simulink model "GhendyanoT2F"  (R2021b)
settings: Solver=ode45  StartTime=0.0  StopTime=TempoSimulacao  RelTol=1e-3  EnableMultiTasking=on
values from neighbouring files (symbols this model uses):
  ccc1 = Ccc*d    [TesteRealCurtoFuses.m]    (also in TesteRealCurto_SemFuse.m)
  ccc2 = Ccc*d    [TesteRealCurtoFuses.m]    (also in TesteRealCurto_SemFuse.m)
  cct1 = Cct*d    [TesteRealCurtoFuses.m]    (also in TesteRealCurto_SemFuse.m)
  cct2 = Cct*d    [TesteRealCurtoFuses.m]    (also in TesteRealCurto_SemFuse.m)
  cequa1 = Ceq*d    [TesteRealCurtoFuses.m]    (also in TesteRealCurto_SemFuse.m)
  cequa2 = Ceq*d    [TesteRealCurtoFuses.m]    (also in TesteRealCurto_SemFuse.m)
  FatorSimulacao = 1e-3    (= 0.001)    [TesteRealCurtoFuses.m]    (also in TesteRealCurto_SemFuse.m)
  le = 1e-10    [TesteRealCurto.m]    (also in TesteRealCurtoFuses.m; TesteRealCurto_SemFuse.m)
  lm1 = lm    [TesteRealCurto.m]    (also in TesteRealCurtoFuses.m; TesteRealCurto_SemFuse.m)
  lm2 = lm    [TesteRealCurto.m]    (also in TesteRealCurtoFuses.m; TesteRealCurto_SemFuse.m)
  lp1 = lp    [TesteRealCurto.m]    (also in TesteRealCurtoFuses.m; TesteRealCurto_SemFuse.m)
  lp2 = lp    [TesteRealCurto.m]    (also in TesteRealCurtoFuses.m; TesteRealCurto_SemFuse.m)
  NRE = 1e-12    [TesteRealCurto.m]    (also in TesteRealCurtoFuses.m; TesteRealCurto_SemFuse.m)
  Raf1 = inf    [TesteRealCurto.m]    (also in TesteRealCurtoFuses.m; TesteRealCurto_SemFuse.m)
  Raf2 = inf    [TesteRealCurto.m]    (also in TesteRealCurtoFuses.m; TesteRealCurto_SemFuse.m)
  Rbf1 = inf    [TesteRealCurto.m]    (also in TesteRealCurtoFuses.m; TesteRealCurto_SemFuse.m)
  Rbf2 = inf    [TesteRealCurto.m]    (also in TesteRealCurtoFuses.m; TesteRealCurto_SemFuse.m)
  Rcf1 = inf    [TesteRealCurto.m]    (also in TesteRealCurtoFuses.m; TesteRealCurto_SemFuse.m)
  Rcf2 = inf    [TesteRealCurto.m]    (also in TesteRealCurtoFuses.m; TesteRealCurto_SemFuse.m)
  rm1 = rm    [TesteRealCurto.m]    (also in TesteRealCurtoFuses.m; TesteRealCurto_SemFuse.m)
  rm2 = rm    [TesteRealCurto.m]    (also in TesteRealCurtoFuses.m; TesteRealCurto_SemFuse.m)
  rp1 = rp    [TesteRealCurto.m]    (also in TesteRealCurtoFuses.m; TesteRealCurto_SemFuse.m)
  rp2 = rp    [TesteRealCurto.m]    (also in TesteRealCurtoFuses.m; TesteRealCurto_SemFuse.m)
  rtc1 = 8    [TesteRealCurto.m]    (also in TesteRealCurtoFuses.m; TesteRealCurto_SemFuse.m)
  rtc2 = 8    [TesteRealCurto.m]    (also in TesteRealCurtoFuses.m; TesteRealCurto_SemFuse.m)
  rti = 10    [TesteRealCurto.m]    (also in TesteRealCurtoFuses.m; TesteRealCurto_SemFuse.m)
undefined symbols (not defined in the file or in its folder): D11, Delta
libraries: spsSeriesRLCBranchLib x26, spsRMSLib x14, spsBreakerLib x9, spsCurrentMeasurementLib x9, spsThreePhaseTransformerTwoWindingsLib x4, spsThreePhaseVIMeasurementLib x3, spsMutualInductanceLib x2, spsThreePhaseSeriesRLCLoadLib x2, spsThreePhaseSourceLib x1, spspowerguiLib x1
(part 2 of 2)

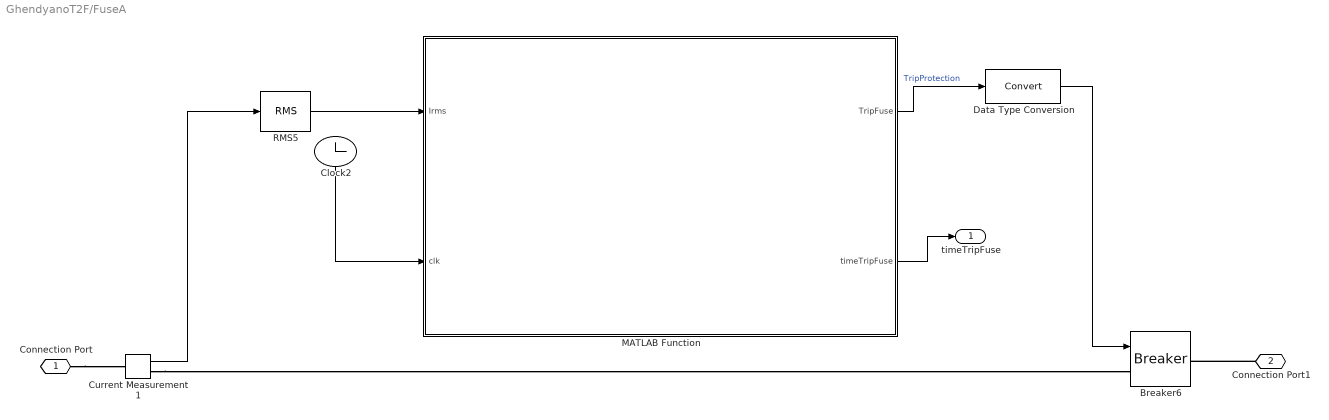
== system GhendyanoT2F/FuseA ==
  Breaker6 : spsBreakerLib/Breaker  InitialState=1  SwitchingTimes="[1/60  5/60]"  External=on  BreakerResistance=0.01  SnubberResistance=1e6  SnubberCapacitance=inf  Measurements=None  MoreParameters=on  NoBreakLoop=off
      settings: SourceProductBaseCode=PS
  Clock2 : Clock
      settings: Decimation=1000
  Current Measurement1 : spsCurrentMeasurementLib/Current Measurement  PhasorSimulation=off  OutputType=Complex  PSBequivalent=0
  Data Type Conversion : DataTypeConversion
  MATLAB Function : MATLAB Function
  RMS5 : spsRMSLib/RMS  TrueRMS=on  Freq=60  RMSInit=0  Ts=0
  Connection Port : PMIOPort  Side=Right
  Connection Port1 : PMIOPort  Port=2  Side=Left
  timeTripFuse : Outport
  wires:
  MATLAB Function/1(TripFuse) -> Data Type Conversion/1  "TripProtection"
  RMS5/1 -> MATLAB Function/1(Irms)
  Data Type Conversion/1 -> Breaker6/1
  Current Measurement1/1 -> RMS5/1
  Clock2/1 -> MATLAB Function/2(clk)
  MATLAB Function/2(timeTripFuse) -> timeTripFuse/1
  connections:
  Current Measurement1/RConn1 -- Breaker6/LConn1
  Connection Port/RConn1 -- Current Measurement1/LConn1
  Connection Port1/RConn1 -- Breaker6/RConn1

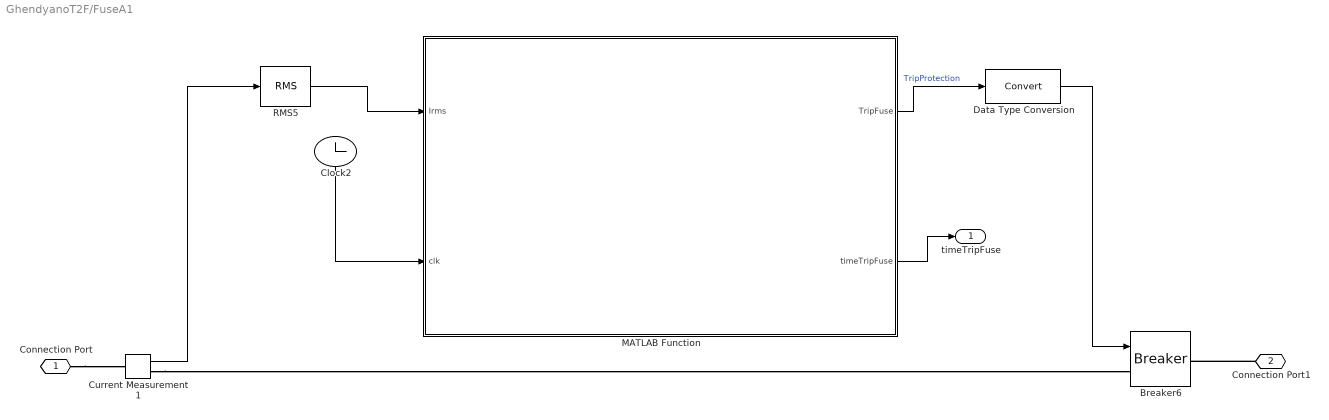
== system GhendyanoT2F/FuseA1 ==
  Breaker6 : spsBreakerLib/Breaker  InitialState=1  SwitchingTimes="[1/60  5/60]"  External=on  BreakerResistance=0.01  SnubberResistance=1e6  SnubberCapacitance=inf  Measurements=None  MoreParameters=on  NoBreakLoop=off
      settings: SourceProductBaseCode=PS
  Clock2 : Clock
      settings: Decimation=1000
  Current Measurement1 : spsCurrentMeasurementLib/Current Measurement  PhasorSimulation=off  OutputType=Complex  PSBequivalent=0
  Data Type Conversion : DataTypeConversion
  MATLAB Function : MATLAB Function
  RMS5 : spsRMSLib/RMS  TrueRMS=on  Freq=60  RMSInit=0  Ts=0
  Connection Port : PMIOPort  Side=Right
  Connection Port1 : PMIOPort  Port=2  Side=Left
  timeTripFuse : Outport
  wires:
  MATLAB Function/1(TripFuse) -> Data Type Conversion/1  "TripProtection"
  RMS5/1 -> MATLAB Function/1(Irms)
  Data Type Conversion/1 -> Breaker6/1
  Current Measurement1/1 -> RMS5/1
  Clock2/1 -> MATLAB Function/2(clk)
  MATLAB Function/2(timeTripFuse) -> timeTripFuse/1
  connections:
  Current Measurement1/RConn1 -- Breaker6/LConn1
  Connection Port/RConn1 -- Current Measurement1/LConn1
  Connection Port1/RConn1 -- Breaker6/RConn1

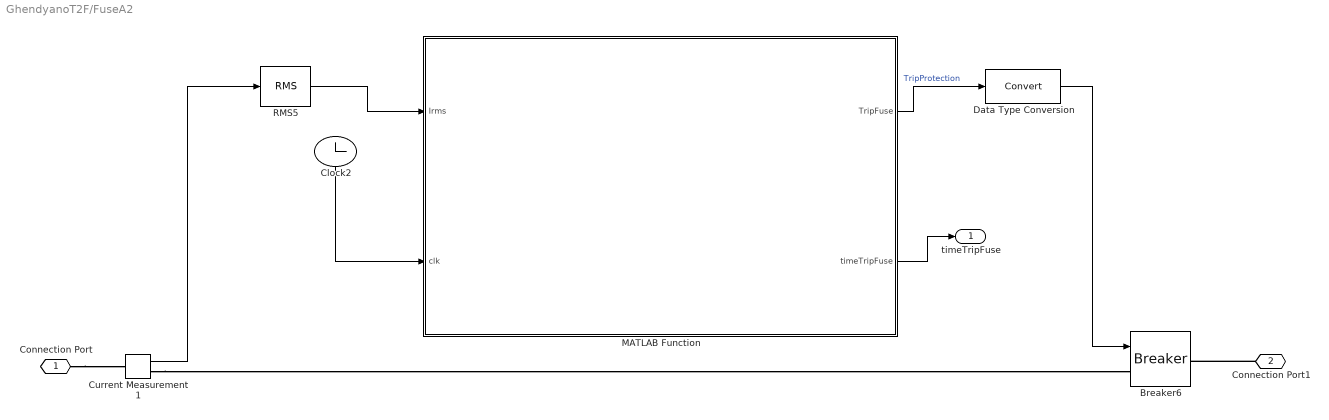
== system GhendyanoT2F/FuseA2 ==
  Breaker6 : spsBreakerLib/Breaker  InitialState=1  SwitchingTimes="[1/60  5/60]"  External=on  BreakerResistance=0.01  SnubberResistance=1e6  SnubberCapacitance=inf  Measurements=None  MoreParameters=on  NoBreakLoop=off
      settings: SourceProductBaseCode=PS
  Clock2 : Clock
      settings: Decimation=1000
  Current Measurement1 : spsCurrentMeasurementLib/Current Measurement  PhasorSimulation=off  OutputType=Complex  PSBequivalent=0
  Data Type Conversion : DataTypeConversion
  MATLAB Function : MATLAB Function
  RMS5 : spsRMSLib/RMS  TrueRMS=on  Freq=60  RMSInit=0  Ts=0
  Connection Port : PMIOPort  Side=Right
  Connection Port1 : PMIOPort  Port=2  Side=Left
  timeTripFuse : Outport
  wires:
  MATLAB Function/1(TripFuse) -> Data Type Conversion/1  "TripProtection"
  RMS5/1 -> MATLAB Function/1(Irms)
  Data Type Conversion/1 -> Breaker6/1
  Current Measurement1/1 -> RMS5/1
  Clock2/1 -> MATLAB Function/2(clk)
  MATLAB Function/2(timeTripFuse) -> timeTripFuse/1
  connections:
  Current Measurement1/RConn1 -- Breaker6/LConn1
  Connection Port/RConn1 -- Current Measurement1/LConn1
  Connection Port1/RConn1 -- Breaker6/RConn1

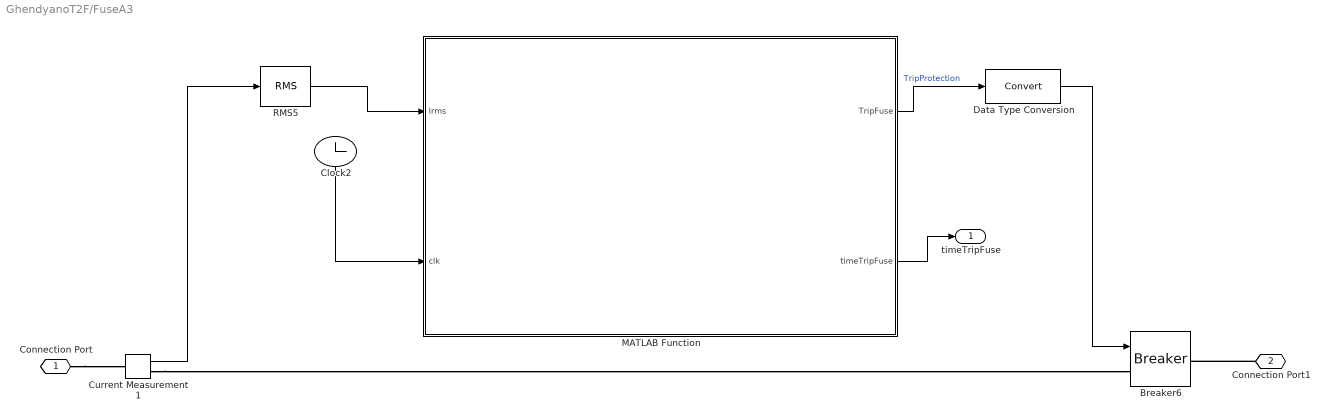
== system GhendyanoT2F/FuseA3 ==
  Breaker6 : spsBreakerLib/Breaker  InitialState=1  SwitchingTimes="[1/60  5/60]"  External=on  BreakerResistance=0.01  SnubberResistance=1e6  SnubberCapacitance=inf  Measurements=None  MoreParameters=on  NoBreakLoop=off
      settings: SourceProductBaseCode=PS
  Clock2 : Clock
      settings: Decimation=1000
  Current Measurement1 : spsCurrentMeasurementLib/Current Measurement  PhasorSimulation=off  OutputType=Complex  PSBequivalent=0
  Data Type Conversion : DataTypeConversion
  MATLAB Function : MATLAB Function
  RMS5 : spsRMSLib/RMS  TrueRMS=on  Freq=60  RMSInit=0  Ts=0
  Connection Port : PMIOPort  Side=Right
  Connection Port1 : PMIOPort  Port=2  Side=Left
  timeTripFuse : Outport
  wires:
  MATLAB Function/1(TripFuse) -> Data Type Conversion/1  "TripProtection"
  RMS5/1 -> MATLAB Function/1(Irms)
  Data Type Conversion/1 -> Breaker6/1
  Current Measurement1/1 -> RMS5/1
  Clock2/1 -> MATLAB Function/2(clk)
  MATLAB Function/2(timeTripFuse) -> timeTripFuse/1
  connections:
  Current Measurement1/RConn1 -- Breaker6/LConn1
  Connection Port/RConn1 -- Current Measurement1/LConn1
  Connection Port1/RConn1 -- Breaker6/RConn1

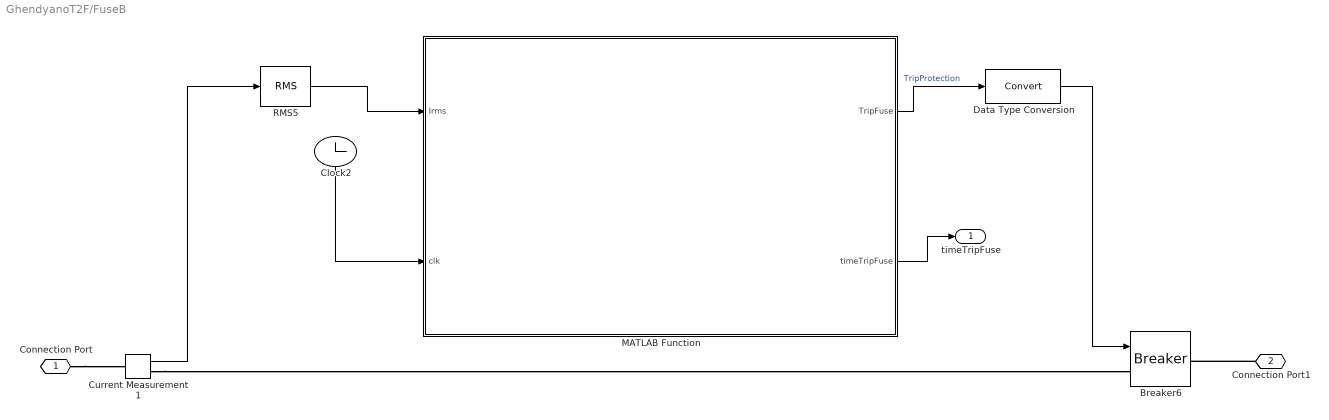
== system GhendyanoT2F/FuseB ==
  Breaker6 : spsBreakerLib/Breaker  InitialState=1  SwitchingTimes="[1/60  5/60]"  External=on  BreakerResistance=0.01  SnubberResistance=1e6  SnubberCapacitance=inf  Measurements=None  MoreParameters=on  NoBreakLoop=off
      settings: SourceProductBaseCode=PS
  Clock2 : Clock
      settings: Decimation=1000
  Current Measurement1 : spsCurrentMeasurementLib/Current Measurement  PhasorSimulation=off  OutputType=Complex  PSBequivalent=0
  Data Type Conversion : DataTypeConversion
  MATLAB Function : MATLAB Function
  RMS5 : spsRMSLib/RMS  TrueRMS=on  Freq=60  RMSInit=0  Ts=0
  Connection Port : PMIOPort  Side=Right
  Connection Port1 : PMIOPort  Port=2  Side=Left
  timeTripFuse : Outport
  wires:
  MATLAB Function/1(TripFuse) -> Data Type Conversion/1  "TripProtection"
  RMS5/1 -> MATLAB Function/1(Irms)
  Data Type Conversion/1 -> Breaker6/1
  Current Measurement1/1 -> RMS5/1
  Clock2/1 -> MATLAB Function/2(clk)
  MATLAB Function/2(timeTripFuse) -> timeTripFuse/1
  connections:
  Current Measurement1/RConn1 -- Breaker6/LConn1
  Connection Port/RConn1 -- Current Measurement1/LConn1
  Connection Port1/RConn1 -- Breaker6/RConn1

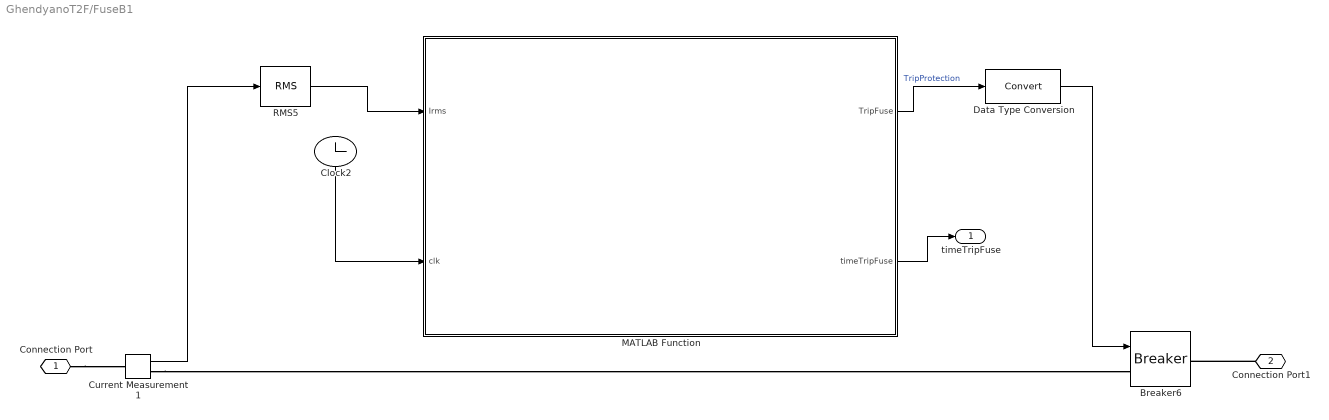
== system GhendyanoT2F/FuseB1 ==
  Breaker6 : spsBreakerLib/Breaker  InitialState=1  SwitchingTimes="[1/60  5/60]"  External=on  BreakerResistance=0.01  SnubberResistance=1e6  SnubberCapacitance=inf  Measurements=None  MoreParameters=on  NoBreakLoop=off
      settings: SourceProductBaseCode=PS
  Clock2 : Clock
      settings: Decimation=1000
  Current Measurement1 : spsCurrentMeasurementLib/Current Measurement  PhasorSimulation=off  OutputType=Complex  PSBequivalent=0
  Data Type Conversion : DataTypeConversion
  MATLAB Function : MATLAB Function
  RMS5 : spsRMSLib/RMS  TrueRMS=on  Freq=60  RMSInit=0  Ts=0
  Connection Port : PMIOPort  Side=Right
  Connection Port1 : PMIOPort  Port=2  Side=Left
  timeTripFuse : Outport
  wires:
  MATLAB Function/1(TripFuse) -> Data Type Conversion/1  "TripProtection"
  RMS5/1 -> MATLAB Function/1(Irms)
  Data Type Conversion/1 -> Breaker6/1
  Current Measurement1/1 -> RMS5/1
  Clock2/1 -> MATLAB Function/2(clk)
  MATLAB Function/2(timeTripFuse) -> timeTripFuse/1
  connections:
  Current Measurement1/RConn1 -- Breaker6/LConn1
  Connection Port/RConn1 -- Current Measurement1/LConn1
  Connection Port1/RConn1 -- Breaker6/RConn1

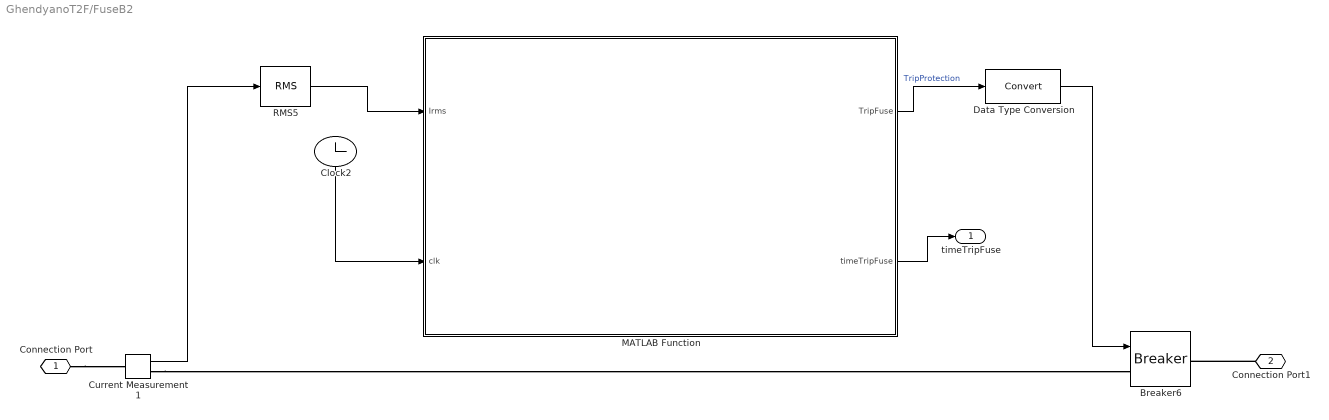
== system GhendyanoT2F/FuseB2 ==
  Breaker6 : spsBreakerLib/Breaker  InitialState=1  SwitchingTimes="[1/60  5/60]"  External=on  BreakerResistance=0.01  SnubberResistance=1e6  SnubberCapacitance=inf  Measurements=None  MoreParameters=on  NoBreakLoop=off
      settings: SourceProductBaseCode=PS
  Clock2 : Clock
      settings: Decimation=1000
  Current Measurement1 : spsCurrentMeasurementLib/Current Measurement  PhasorSimulation=off  OutputType=Complex  PSBequivalent=0
  Data Type Conversion : DataTypeConversion
  MATLAB Function : MATLAB Function
  RMS5 : spsRMSLib/RMS  TrueRMS=on  Freq=60  RMSInit=0  Ts=0
  Connection Port : PMIOPort  Side=Right
  Connection Port1 : PMIOPort  Port=2  Side=Left
  timeTripFuse : Outport
  wires:
  MATLAB Function/1(TripFuse) -> Data Type Conversion/1  "TripProtection"
  RMS5/1 -> MATLAB Function/1(Irms)
  Data Type Conversion/1 -> Breaker6/1
  Current Measurement1/1 -> RMS5/1
  Clock2/1 -> MATLAB Function/2(clk)
  MATLAB Function/2(timeTripFuse) -> timeTripFuse/1
  connections:
  Current Measurement1/RConn1 -- Breaker6/LConn1
  Connection Port/RConn1 -- Current Measurement1/LConn1
  Connection Port1/RConn1 -- Breaker6/RConn1

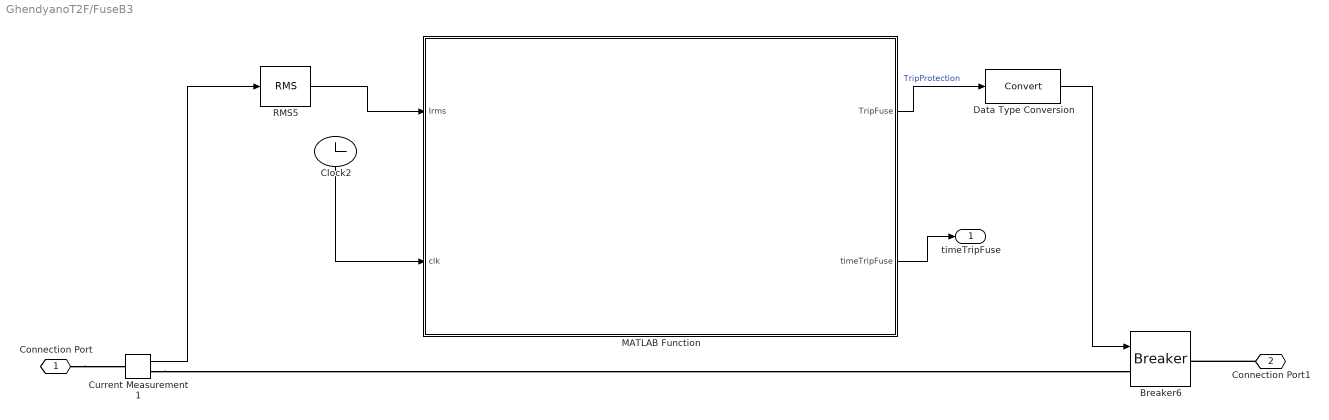
== system GhendyanoT2F/FuseB3 ==
  Breaker6 : spsBreakerLib/Breaker  InitialState=1  SwitchingTimes="[1/60  5/60]"  External=on  BreakerResistance=0.01  SnubberResistance=1e6  SnubberCapacitance=inf  Measurements=None  MoreParameters=on  NoBreakLoop=off
      settings: SourceProductBaseCode=PS
  Clock2 : Clock
      settings: Decimation=1000
  Current Measurement1 : spsCurrentMeasurementLib/Current Measurement  PhasorSimulation=off  OutputType=Complex  PSBequivalent=0
  Data Type Conversion : DataTypeConversion
  MATLAB Function : MATLAB Function
  RMS5 : spsRMSLib/RMS  TrueRMS=on  Freq=60  RMSInit=0  Ts=0
  Connection Port : PMIOPort  Side=Right
  Connection Port1 : PMIOPort  Port=2  Side=Left
  timeTripFuse : Outport
  wires:
  MATLAB Function/1(TripFuse) -> Data Type Conversion/1  "TripProtection"
  RMS5/1 -> MATLAB Function/1(Irms)
  Data Type Conversion/1 -> Breaker6/1
  Current Measurement1/1 -> RMS5/1
  Clock2/1 -> MATLAB Function/2(clk)
  MATLAB Function/2(timeTripFuse) -> timeTripFuse/1
  connections:
  Current Measurement1/RConn1 -- Breaker6/LConn1
  Connection Port/RConn1 -- Current Measurement1/LConn1
  Connection Port1/RConn1 -- Breaker6/RConn1

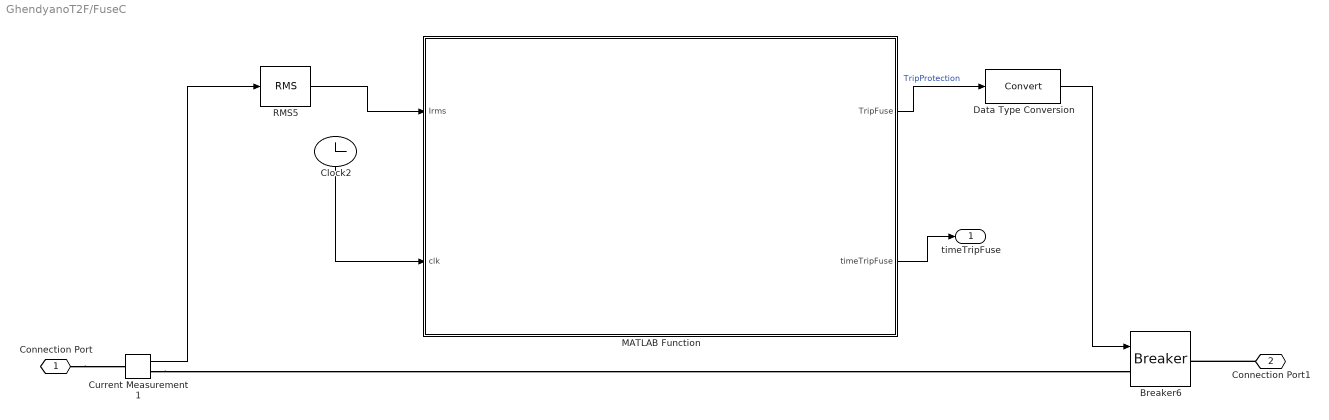
== system GhendyanoT2F/FuseC ==
  Breaker6 : spsBreakerLib/Breaker  InitialState=1  SwitchingTimes="[1/60  5/60]"  External=on  BreakerResistance=0.01  SnubberResistance=1e6  SnubberCapacitance=inf  Measurements=None  MoreParameters=on  NoBreakLoop=off
      settings: SourceProductBaseCode=PS
  Clock2 : Clock
      settings: Decimation=1000
  Current Measurement1 : spsCurrentMeasurementLib/Current Measurement  PhasorSimulation=off  OutputType=Complex  PSBequivalent=0
  Data Type Conversion : DataTypeConversion
  MATLAB Function : MATLAB Function
  RMS5 : spsRMSLib/RMS  TrueRMS=on  Freq=60  RMSInit=0  Ts=0
  Connection Port : PMIOPort  Side=Right
  Connection Port1 : PMIOPort  Port=2  Side=Left
  timeTripFuse : Outport
  wires:
  MATLAB Function/1(TripFuse) -> Data Type Conversion/1  "TripProtection"
  RMS5/1 -> MATLAB Function/1(Irms)
  Data Type Conversion/1 -> Breaker6/1
  Current Measurement1/1 -> RMS5/1
  Clock2/1 -> MATLAB Function/2(clk)
  MATLAB Function/2(timeTripFuse) -> timeTripFuse/1
  connections:
  Current Measurement1/RConn1 -- Breaker6/LConn1
  Connection Port/RConn1 -- Current Measurement1/LConn1
  Connection Port1/RConn1 -- Breaker6/RConn1

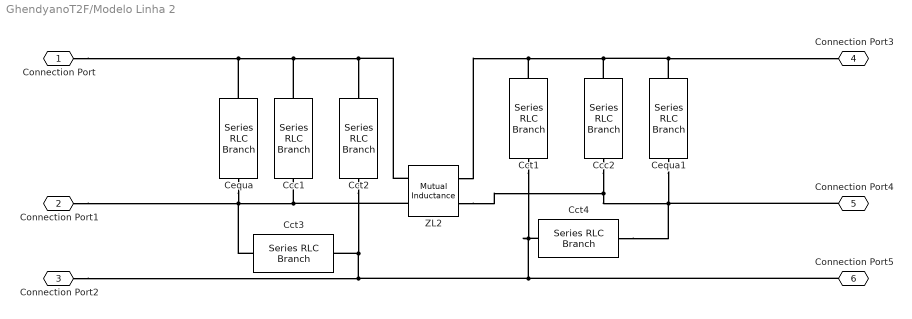
== system GhendyanoT2F/Modelo Linha 2 ==
  Ccc1 : spsSeriesRLCBranchLib/Series RLC Branch  LConnTagsString=__new0  RConnTagsString=__new0  BranchType=C  Resistance=1  Inductance=1e-3  SetiL0=off  InitialCurrent=0  Capacitance=ccc2/2  Setx0=off  InitialVoltage=0  Measurements=Branch voltage
  Ccc2 : spsSeriesRLCBranchLib/Series RLC Branch  LConnTagsString=__new0  RConnTagsString=__new0  BranchType=C  Resistance=1  Inductance=1e-3  SetiL0=off  InitialCurrent=0  Capacitance=ccc2/2  Setx0=off  InitialVoltage=0  Measurements=Branch voltage
  Cct{1..4} (4 alike) : spsSeriesRLCBranchLib/Series RLC Branch  LConnTagsString=__new0  RConnTagsString=__new0  BranchType=C  Resistance=1  Inductance=1e-3  SetiL0=off  InitialCurrent=0  Capacitance=cct2/2  Setx0=off  InitialVoltage=0  Measurements=None
  Cequa : spsSeriesRLCBranchLib/Series RLC Branch  LConnTagsString=__new0  RConnTagsString=__new0  BranchType=C  Resistance=1  Inductance=1e-3  SetiL0=off  InitialCurrent=0  Capacitance=cequa2/2  Setx0=off  InitialVoltage=0  Measurements=None
  Cequa1 : spsSeriesRLCBranchLib/Series RLC Branch  LConnTagsString=__new0  RConnTagsString=__new0  BranchType=C  Resistance=1  Inductance=1e-3  SetiL0=off  InitialCurrent=0  Capacitance=cequa2/2  Setx0=off  InitialVoltage=0  Measurements=None
  ZL2 : spsMutualInductanceLib/Mutual Inductance  LConnTagsString=a|b  RConnTagsString=A|B  TypeOfMutual=Generalized mutual inductance  NumberOfWindings=2  SelfImpedance1=[1.1 1.1e-03]  SelfImpedance2=[ 1.1 1.1e-03]  ThreeWindings=on  SelfImpedance3=[ 1.1 1.1e-03]  MutualImpedance=[1.0 1.0e-03]  InductanceMatrix=[lp2 lm2 ; lm2 lp2]  ResistanceMatrix=[rp2 rm2 ; rm2 rp2]  Measurements=None
      settings: SourceProductBaseCode=PS
  Connection Port : PMIOPort  Side=Left
  Connection Port1 : PMIOPort  Port=2  Side=Left
  Connection Port2 : PMIOPort  Port=3  Side=Left
  Connection Port3 : PMIOPort  Port=4  Side=Right
  Connection Port4 : PMIOPort  Port=5  Side=Right
  Connection Port5 : PMIOPort  Port=6  Side=Right
  connections:
  Ccc1/LConn1 -- Cequa/LConn1 -- Connection Port/RConn1 -- ZL2/LConn1 -- Cct2/LConn1
  Cct3/LConn1 -- ZL2/LConn2 -- Ccc1/RConn1 -- Cequa/RConn1 -- Connection Port1/RConn1
  Cct1/RConn1 -- Cct4/LConn1 -- Connection Port5/RConn1 -- Connection Port2/RConn1 -- Cct2/RConn1 -- Cct3/RConn1
  Connection Port4/RConn1 -- ZL2/RConn2 -- Ccc2/RConn1 -- Cequa1/RConn1 -- Cct4/RConn1
  Cequa1/LConn1 -- ZL2/RConn1 -- Cct1/LConn1 -- Ccc2/LConn1 -- Connection Port3/RConn1

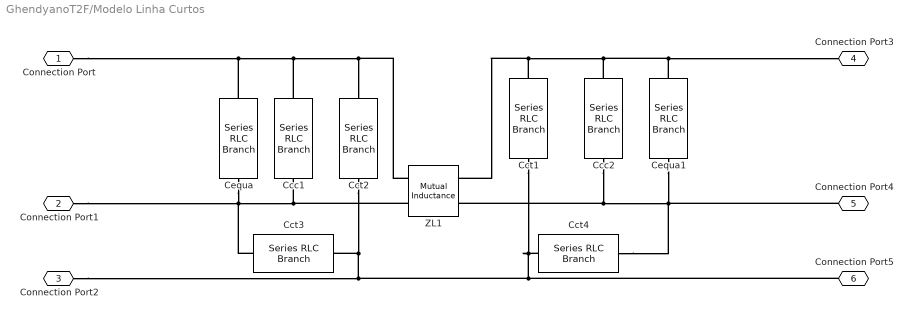
== system GhendyanoT2F/Modelo Linha Curtos ==
  Ccc1 : spsSeriesRLCBranchLib/Series RLC Branch  LConnTagsString=__new0  RConnTagsString=__new0  BranchType=C  Resistance=1  Inductance=1e-3  SetiL0=off  InitialCurrent=0  Capacitance=ccc1/2  Setx0=off  InitialVoltage=0  Measurements=Branch voltage
  Ccc2 : spsSeriesRLCBranchLib/Series RLC Branch  LConnTagsString=__new0  RConnTagsString=__new0  BranchType=C  Resistance=1  Inductance=1e-3  SetiL0=off  InitialCurrent=0  Capacitance=ccc1/2  Setx0=off  InitialVoltage=0  Measurements=Branch voltage
  Cct{1..4} (4 alike) : spsSeriesRLCBranchLib/Series RLC Branch  LConnTagsString=__new0  RConnTagsString=__new0  BranchType=C  Resistance=1  Inductance=1e-3  SetiL0=off  InitialCurrent=0  Capacitance=cct1/2  Setx0=off  InitialVoltage=0  Measurements=None
  Cequa : spsSeriesRLCBranchLib/Series RLC Branch  LConnTagsString=__new0  RConnTagsString=__new0  BranchType=C  Resistance=1  Inductance=1e-3  SetiL0=off  InitialCurrent=0  Capacitance=cequa1/2  Setx0=off  InitialVoltage=0  Measurements=None
  Cequa1 : spsSeriesRLCBranchLib/Series RLC Branch  LConnTagsString=__new0  RConnTagsString=__new0  BranchType=C  Resistance=1  Inductance=1e-3  SetiL0=off  InitialCurrent=0  Capacitance=cequa1/2  Setx0=off  InitialVoltage=0  Measurements=None
  ZL1 : spsMutualInductanceLib/Mutual Inductance  LConnTagsString=a|b  RConnTagsString=A|B  TypeOfMutual=Generalized mutual inductance  NumberOfWindings=2  SelfImpedance1=[1.1 1.1e-03]  SelfImpedance2=[ 1.1 1.1e-03]  ThreeWindings=on  SelfImpedance3=[ 1.1 1.1e-03]  MutualImpedance=[1.0 1.0e-03]  InductanceMatrix=[lp1 lm1 ; lm1 lp1]  ResistanceMatrix=[rp1 rm1 ; rm1 rp1]  Measurements=None
      settings: SourceProductBaseCode=PS
  Connection Port : PMIOPort  Side=Left
  Connection Port1 : PMIOPort  Port=2  Side=Left
  Connection Port2 : PMIOPort  Port=3  Side=Left
  Connection Port3 : PMIOPort  Port=4  Side=Right
  Connection Port4 : PMIOPort  Port=5  Side=Right
  Connection Port5 : PMIOPort  Port=6  Side=Right
  connections:
  ZL1/LConn1 -- Cct2/LConn1 -- Ccc1/LConn1 -- Cequa/LConn1 -- Connection Port/RConn1
  ZL1/LConn2 -- Connection Port1/RConn1 -- Cct3/LConn1 -- Cequa/RConn1 -- Ccc1/RConn1
  Cct2/RConn1 -- Cct1/RConn1 -- Cct4/LConn1 -- Connection Port5/RConn1 -- Connection Port2/RConn1 -- Cct3/RConn1
  Connection Port4/RConn1 -- Cequa1/RConn1 -- Ccc2/RConn1 -- ZL1/RConn2 -- Cct4/RConn1
  Cequa1/LConn1 -- Connection Port3/RConn1 -- Cct1/LConn1 -- ZL1/RConn1 -- Ccc2/LConn1

== matlab function GhendyanoT2F/FuseB1/MATLAB Function ==
  settings: updateMethod=DISCRETE
  data: Irms input; clk input; TripFuse output; a parameter; b parameter; c parameter; d parameter; e parameter; timeTripFuse output; IoTot parameter
function [TripFuse, timeTripFuse ]  =  fcn(Irms, clk, a, b, c, d, e, IoTot)
persistent RelayStateOvercurrentTime OperatingTime PickupTime TripTime signal valorIRMS y t timeTrip ValorAbertura
if isempty(RelayStateOvercurrentTime)
    RelayStateOvercurrentTime = 0;
    TripTime = 0;
    signal = 1;
    OperatingTime = inf;
    PickupTime = 0;
    valorIRMS = 0;
    timeTrip = inf;
    ValorAbertura = inf;
end

%% tripFuse
if (RelayStateOvercurrentTime == 0)&&(Irms > IoTot*3)
    PickupTime = clk+0.07;
    RelayStateOvercurrentTime = 1;
end

if(RelayStateOvercurrentTime == 1)&&(clk>PickupTime)
    valorIRMS = Irms;
    y = log(valorIRMS);
    t = a + (b * y) + (c * y^2) + (d * y^3) + (e * y^4);
    OperatingTime = exp(t);
    TripTime = PickupTime + OperatingTime;
    RelayStateOvercurrentTime = 2;
end

if (clk > TripTime)&&(RelayStateOvercurrentTime == 2)
    if ((Irms <= valorIRMS*0.5)&&(Irms <= IoTot*3))
        signal = 1;
        RelayStateOvercurrentTime = 0;
        TripTime = inf;
    else
        ValorAbertura = clk;
        signal = 0;
        RelayStateOvercurrentTime = 3;
        timeTrip = OperatingTime;
    end
end

TripFuse = signal;
timeTripFuse = [valorIRMS timeTrip ValorAbertura];

== matlab function GhendyanoT2F/FuseA3/MATLAB Function ==
  settings: updateMethod=DISCRETE
  data: Irms input; clk input; TripFuse output; a parameter; b parameter; c parameter; d parameter; e parameter; timeTripFuse output; IoTot parameter
function [TripFuse, timeTripFuse ]  =  fcn(Irms, clk, a, b, c, d, e, IoTot)
persistent RelayStateOvercurrentTime OperatingTime PickupTime TripTime signal valorIRMS y t timeTrip ValorAbertura
if isempty(RelayStateOvercurrentTime)
    RelayStateOvercurrentTime = 0;
    TripTime = 0;
    signal = 1;
    OperatingTime = inf;
    PickupTime = 0;
    valorIRMS = 0;
    timeTrip = inf;
    ValorAbertura = inf;
end

%% tripFuse
if (RelayStateOvercurrentTime == 0)&&(Irms > IoTot*3)
    PickupTime = clk+0.07;
    RelayStateOvercurrentTime = 1;
end

if(RelayStateOvercurrentTime == 1)&&(clk>PickupTime)
    valorIRMS = Irms;
    y = log(valorIRMS);
    t = a + (b * y) + (c * y^2) + (d * y^3) + (e * y^4);
    OperatingTime = exp(t);
    TripTime = PickupTime + OperatingTime;
    RelayStateOvercurrentTime = 2;
end

if (clk > TripTime)&&(RelayStateOvercurrentTime == 2)
    if ((Irms <= valorIRMS*0.5)&&(Irms <= IoTot*3))
        signal = 1;
        RelayStateOvercurrentTime = 0;
        TripTime = inf;
    else
        ValorAbertura = clk;
        signal = 0;
        RelayStateOvercurrentTime = 3;
        timeTrip = OperatingTime;
    end
end

TripFuse = signal;
timeTripFuse = [valorIRMS timeTrip ValorAbertura];

== matlab function GhendyanoT2F/FuseB3/MATLAB Function ==
  settings: updateMethod=DISCRETE
  data: Irms input; clk input; TripFuse output; a parameter; b parameter; c parameter; d parameter; e parameter; timeTripFuse output; IoTot parameter
function [TripFuse, timeTripFuse ]  =  fcn(Irms, clk, a, b, c, d, e, IoTot)
persistent RelayStateOvercurrentTime OperatingTime PickupTime TripTime signal valorIRMS y t timeTrip ValorAbertura
if isempty(RelayStateOvercurrentTime)
    RelayStateOvercurrentTime = 0;
    TripTime = 0;
    signal = 1;
    OperatingTime = inf;
    PickupTime = 0;
    valorIRMS = 0;
    timeTrip = inf;
    ValorAbertura = inf;
end

%% tripFuse
if (RelayStateOvercurrentTime == 0)&&(Irms > IoTot*3)
    PickupTime = clk+0.07;
    RelayStateOvercurrentTime = 1;
end

if(RelayStateOvercurrentTime == 1)&&(clk>PickupTime)
    valorIRMS = Irms;
    y = log(valorIRMS);
    t = a + (b * y) + (c * y^2) + (d * y^3) + (e * y^4);
    OperatingTime = exp(t);
    TripTime = PickupTime + OperatingTime;
    RelayStateOvercurrentTime = 2;
end

if (clk > TripTime)&&(RelayStateOvercurrentTime == 2)
    if ((Irms <= valorIRMS*0.5)&&(Irms <= IoTot*3))
        signal = 1;
        RelayStateOvercurrentTime = 0;
        TripTime = inf;
    else
        ValorAbertura = clk;
        signal = 0;
        RelayStateOvercurrentTime = 3;
        timeTrip = OperatingTime;
    end
end

TripFuse = signal;
timeTripFuse = [valorIRMS timeTrip ValorAbertura];

== matlab function GhendyanoT2F/FuseA/MATLAB Function ==
  settings: updateMethod=DISCRETE
  data: Irms input; clk input; TripFuse output; a parameter; b parameter; c parameter; d parameter; e parameter; timeTripFuse output; IoTot parameter
function [TripFuse, timeTripFuse ]  =  fcn(Irms, clk, a, b, c, d, e, IoTot)
persistent RelayStateOvercurrentTime OperatingTime PickupTime TripTime signal valorIRMS y t timeTrip ValorAbertura
if isempty(RelayStateOvercurrentTime)
    RelayStateOvercurrentTime = 0;
    TripTime = 0;
    signal = 1;
    OperatingTime = inf;
    PickupTime = 0;
    valorIRMS = 0;
    timeTrip = inf;
    ValorAbertura = inf;
end

%% tripFuse
if (RelayStateOvercurrentTime == 0)&&(Irms > IoTot*3)
    PickupTime = clk+0.07;
    RelayStateOvercurrentTime = 1;
end

if(RelayStateOvercurrentTime == 1)&&(clk>PickupTime)
    valorIRMS = Irms;
    y = log(valorIRMS);
    t = a + (b * y) + (c * y^2) + (d * y^3) + (e * y^4);
    OperatingTime = exp(t);
    TripTime = PickupTime + OperatingTime;
    RelayStateOvercurrentTime = 2;
end

if (clk > TripTime)&&(RelayStateOvercurrentTime == 2)
    if ((Irms <= valorIRMS*0.5)&&(Irms <= IoTot*3))
        signal = 1;
        RelayStateOvercurrentTime = 0;
        TripTime = inf;
    else
        ValorAbertura = clk;
        signal = 0;
        RelayStateOvercurrentTime = 3;
        timeTrip = OperatingTime;
    end
end

TripFuse = signal;
timeTripFuse = [valorIRMS timeTrip ValorAbertura];

== matlab function GhendyanoT2F/FuseB/MATLAB Function ==
  settings: updateMethod=DISCRETE
  data: Irms input; clk input; TripFuse output; a parameter; b parameter; c parameter; d parameter; e parameter; timeTripFuse output; IoTot parameter
function [TripFuse, timeTripFuse ]  =  fcn(Irms, clk, a, b, c, d, e, IoTot)
persistent RelayStateOvercurrentTime OperatingTime PickupTime TripTime signal valorIRMS y t timeTrip ValorAbertura
if isempty(RelayStateOvercurrentTime)
    RelayStateOvercurrentTime = 0;
    TripTime = 0;
    signal = 1;
    OperatingTime = inf;
    PickupTime = 0;
    valorIRMS = 0;
    timeTrip = inf;
    ValorAbertura = inf;
end

%% tripFuse
if (RelayStateOvercurrentTime == 0)&&(Irms > IoTot*3)
    PickupTime = clk+0.07;
    RelayStateOvercurrentTime = 1;
end

if(RelayStateOvercurrentTime == 1)&&(clk>PickupTime)
    valorIRMS = Irms;
    y = log(valorIRMS);
    t = a + (b * y) + (c * y^2) + (d * y^3) + (e * y^4);
    OperatingTime = exp(t);
    TripTime = PickupTime + OperatingTime;
    RelayStateOvercurrentTime = 2;
end

if (clk > TripTime)&&(RelayStateOvercurrentTime == 2)
    if ((Irms <= valorIRMS*0.5)&&(Irms <= IoTot*3))
        signal = 1;
        RelayStateOvercurrentTime = 0;
        TripTime = inf;
    else
        ValorAbertura = clk;
        signal = 0;
        RelayStateOvercurrentTime = 3;
        timeTrip = OperatingTime;
    end
end

TripFuse = signal;
timeTripFuse = [valorIRMS timeTrip ValorAbertura];

== matlab function GhendyanoT2F/FuseC/MATLAB Function ==
  settings: updateMethod=DISCRETE
  data: Irms input; clk input; TripFuse output; a parameter; b parameter; c parameter; d parameter; e parameter; timeTripFuse output; IoTot parameter
function [TripFuse, timeTripFuse ]  =  fcn(Irms, clk, a, b, c, d, e, IoTot)
persistent RelayStateOvercurrentTime OperatingTime PickupTime TripTime signal valorIRMS y t timeTrip ValorAbertura
if isempty(RelayStateOvercurrentTime)
    RelayStateOvercurrentTime = 0;
    TripTime = 0;
    signal = 1;
    OperatingTime = inf;
    PickupTime = 0;
    valorIRMS = 0;
    timeTrip = inf;
    ValorAbertura = inf;
end

%% tripFuse
if (RelayStateOvercurrentTime == 0)&&(Irms > IoTot*3)
    PickupTime = clk+0.07;
    RelayStateOvercurrentTime = 1;
end

if(RelayStateOvercurrentTime == 1)&&(clk>PickupTime)
    valorIRMS = Irms;
    y = log(valorIRMS);
    t = a + (b * y) + (c * y^2) + (d * y^3) + (e * y^4);
    OperatingTime = exp(t);
    TripTime = PickupTime + OperatingTime;
    RelayStateOvercurrentTime = 2;
end

if (clk > TripTime)&&(RelayStateOvercurrentTime == 2)
    if ((Irms <= valorIRMS*0.5)&&(Irms <= IoTot*3))
        signal = 1;
        RelayStateOvercurrentTime = 0;
        TripTime = inf;
    else
        ValorAbertura = clk;
        signal = 0;
        RelayStateOvercurrentTime = 3;
        timeTrip = OperatingTime;
    end
end

TripFuse = signal;
timeTripFuse = [valorIRMS timeTrip ValorAbertura];

== matlab function GhendyanoT2F/FuseA2/MATLAB Function ==
  settings: updateMethod=DISCRETE
  data: Irms input; clk input; TripFuse output; a parameter; b parameter; c parameter; d parameter; e parameter; timeTripFuse output; IoTot parameter
function [TripFuse, timeTripFuse ]  =  fcn(Irms, clk, a, b, c, d, e, IoTot)
persistent RelayStateOvercurrentTime OperatingTime PickupTime TripTime signal valorIRMS y t timeTrip ValorAbertura
if isempty(RelayStateOvercurrentTime)
    RelayStateOvercurrentTime = 0;
    TripTime = 0;
    signal = 1;
    OperatingTime = inf;
    PickupTime = 0;
    valorIRMS = 0;
    timeTrip = inf;
    ValorAbertura = inf;
end

%% tripFuse
if (RelayStateOvercurrentTime == 0)&&(Irms > IoTot*3)
    PickupTime = clk+0.07;
    RelayStateOvercurrentTime = 1;
end

if(RelayStateOvercurrentTime == 1)&&(clk>PickupTime)
    valorIRMS = Irms;
    y = log(valorIRMS);
    t = a + (b * y) + (c * y^2) + (d * y^3) + (e * y^4);
    OperatingTime = exp(t);
    TripTime = PickupTime + OperatingTime;
    RelayStateOvercurrentTime = 2;
end

if (clk > TripTime)&&(RelayStateOvercurrentTime == 2)
    if ((Irms <= valorIRMS*0.5)&&(Irms <= IoTot*3))
        signal = 1;
        RelayStateOvercurrentTime = 0;
        TripTime = inf;
    else
        ValorAbertura = clk;
        signal = 0;
        RelayStateOvercurrentTime = 3;
        timeTrip = OperatingTime;
    end
end

TripFuse = signal;
timeTripFuse = [valorIRMS timeTrip ValorAbertura];

== matlab function GhendyanoT2F/FuseB2/MATLAB Function ==
  settings: updateMethod=DISCRETE
  data: Irms input; clk input; TripFuse output; a parameter; b parameter; c parameter; d parameter; e parameter; timeTripFuse output; IoTot parameter
function [TripFuse, timeTripFuse ]  =  fcn(Irms, clk, a, b, c, d, e, IoTot)
persistent RelayStateOvercurrentTime OperatingTime PickupTime TripTime signal valorIRMS y t timeTrip ValorAbertura
if isempty(RelayStateOvercurrentTime)
    RelayStateOvercurrentTime = 0;
    TripTime = 0;
    signal = 1;
    OperatingTime = inf;
    PickupTime = 0;
    valorIRMS = 0;
    timeTrip = inf;
    ValorAbertura = inf;
end

%% tripFuse
if (RelayStateOvercurrentTime == 0)&&(Irms > IoTot*3)
    PickupTime = clk+0.07;
    RelayStateOvercurrentTime = 1;
end

if(RelayStateOvercurrentTime == 1)&&(clk>PickupTime)
    valorIRMS = Irms;
    y = log(valorIRMS);
    t = a + (b * y) + (c * y^2) + (d * y^3) + (e * y^4);
    OperatingTime = exp(t);
    TripTime = PickupTime + OperatingTime;
    RelayStateOvercurrentTime = 2;
end

if (clk > TripTime)&&(RelayStateOvercurrentTime == 2)
    if ((Irms <= valorIRMS*0.5)&&(Irms <= IoTot*3))
        signal = 1;
        RelayStateOvercurrentTime = 0;
        TripTime = inf;
    else
        ValorAbertura = clk;
        signal = 0;
        RelayStateOvercurrentTime = 3;
        timeTrip = OperatingTime;
    end
end

TripFuse = signal;
timeTripFuse = [valorIRMS timeTrip ValorAbertura];

== matlab function GhendyanoT2F/FuseA1/MATLAB Function ==
  settings: updateMethod=DISCRETE
  data: Irms input; clk input; TripFuse output; a parameter; b parameter; c parameter; d parameter; e parameter; timeTripFuse output; IoTot parameter
function [TripFuse, timeTripFuse ]  =  fcn(Irms, clk, a, b, c, d, e, IoTot)
persistent RelayStateOvercurrentTime OperatingTime PickupTime TripTime signal valorIRMS y t timeTrip ValorAbertura
if isempty(RelayStateOvercurrentTime)
    RelayStateOvercurrentTime = 0;
    TripTime = 0;
    signal = 1;
    OperatingTime = inf;
    PickupTime = 0;
    valorIRMS = 0;
    timeTrip = inf;
    ValorAbertura = inf;
end

%% tripFuse
if (RelayStateOvercurrentTime == 0)&&(Irms > IoTot*3)
    PickupTime = clk+0.07;
    RelayStateOvercurrentTime = 1;
end

if(RelayStateOvercurrentTime == 1)&&(clk>PickupTime)
    valorIRMS = Irms;
    y = log(valorIRMS);
    t = a + (b * y) + (c * y^2) + (d * y^3) + (e * y^4);
    OperatingTime = exp(t);
    TripTime = PickupTime + OperatingTime;
    RelayStateOvercurrentTime = 2;
end

if (clk > TripTime)&&(RelayStateOvercurrentTime == 2)
    if ((Irms <= valorIRMS*0.5)&&(Irms <= IoTot*3))
        signal = 1;
        RelayStateOvercurrentTime = 0;
        TripTime = inf;
    else
        ValorAbertura = clk;
        signal = 0;
        RelayStateOvercurrentTime = 3;
        timeTrip = OperatingTime;
    end
end

TripFuse = signal;
timeTripFuse = [valorIRMS timeTrip ValorAbertura];
